simulink model "Lab03_LTI-viewer"  (R2021b)
settings: Solver=ode45  StartTime=0.0  StopTime=10.0  RelTol=1e-3  EnableMultiTasking=on
settings Model: Creator=User_Admin  LastModifiedBy=User_Admin
settings DataIOCC: LimitDataPoints=on  SaveFormat=Array  SignalLoggingSaveFormat=ModelDataLogs  ReturnWorkspaceOutputs=off
settings OptimizationCC: BooleanDataType=off
settings DebuggingCC: SaveWithParameterizedLinksMsg=none  UnderspecifiedInitializationDetection=Classic  MergeDetectMultiDrivingBlocksExec=none  SignalResolutionControl=TryResolveAllWithWarning  MultiTaskDSMMsg=warning  MultiTaskCondExecSysMsg=none
settings HardwareCC: TargetUnknown=on
settings ModelReferenceCC: PropagateSignalLabelsOutOfModel=off
settings GRTTargetCC: CombineOutputUpdateFcns=off  GRTInterface=on
settings ConfigComp: CovMetricSettings=dw

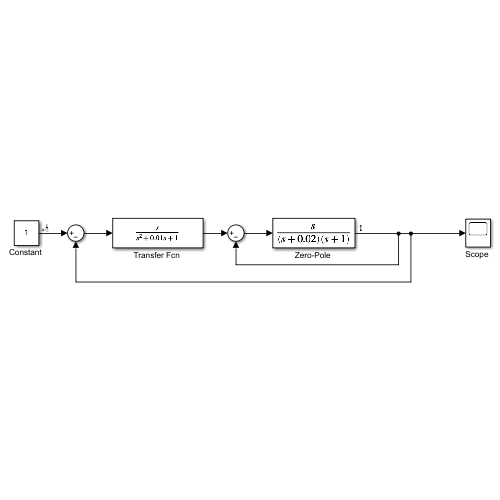
[thumbnail: Simulink's stored preview of the top-level diagram]
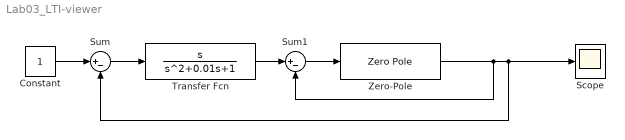
== system Lab03_LTI-viewer ==
  "Constant " : Constant
  "Scope " : Scope
  Sum : Sum  Inputs=|+-  SaturateOnIntegerOverflow=on
  Sum1 : Sum  Inputs=|+-  SaturateOnIntegerOverflow=on
  "Transfer Fcn " : TransferFcn  Numerator=[1 0]  Denominator=[1 0.01 1]
  "Zero-Pole " : ZeroPole  Zeros=[0]  Poles=[-0.02 -1]
  wires:
  Sum/1 -> "Transfer Fcn "/1
  "Transfer Fcn "/1 -> Sum1/1
  Sum1/1 -> "Zero-Pole "/1
  "Zero-Pole "/1 -> Sum1/2, Sum/2, "Scope "/1
  "Constant "/1 -> Sum/1
